simulink model "DCMotorControl"  (R2024b)
settings: Solver=VariableStepAuto  StartTime=0.0  StopTime=2  RelTol=1e-3
libraries: slpidlib x1
settings Model: Creator=chenitzhak6  LastModifiedBy=lenovo

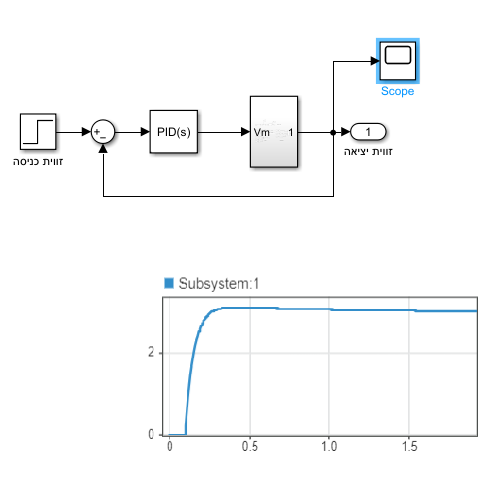
[thumbnail: Simulink's stored preview of the top-level diagram]
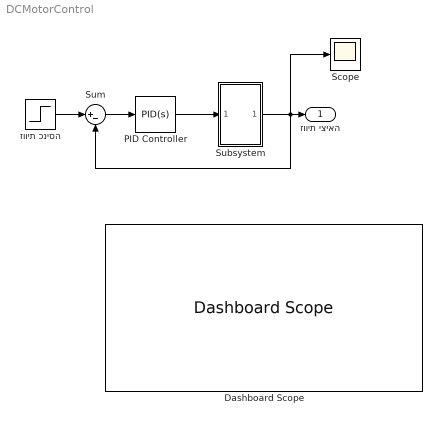
== system DCMotorControl ==
  Dashboard Scope : DashboardScope
  PID Controller : slpidlib/PID Controller  Controller=PID  Form=Parallel  TimeDomain=Continuous-time  UseExternalTs=off  SampleTime=-1  IntegratorMethod=Forward Euler  FilterMethod=Forward Euler  ControllerParametersSource=internal  P=1  I=1  UseKiTs=off  D=0  UseExternalDerivativeSource=off  N=100  UseFilter=on  TunerSelectOption=Transfer Function Based (PID Tuner App)  InitialConditionSource=internal  InitialConditionForIntegrator=0  InitialConditionForFilter=0  DifferentiatorICPrevScaledInput=0  ExternalReset=none  TrackingMode=off  Kt=1  LimitOutput=off  SatLimitsSource=internal  UpperSaturationLimit=inf  LowerSaturationLimit=-inf  LinearizeAsGain=on  AntiWindupMode=none  Kb=1  LimitIntegrator=off  UpperIntegratorSaturationLimit=inf  LowerIntegratorSaturationLimit=-inf  POutMin=[]  POutMax=[]  IOutMin=[]  IOutMax=[]  DOutMin=[]  DOutMax=[]  NOutMin=[]  NOutMax=[]  SumOutMin=[]  SumOutMax=[]  SaturationOutMin=[]  SaturationOutMax=[]  PParamMin=[]  PParamMax=[]  IParamMin=[]  IParamMax=[]  DParamMin=[]  DParamMax=[]  NParamMin=[]  NParamMax=[]  KbParamMin=[]  KbParamMax=[]  KtParamMin=[]  KtParamMax=[]  KbOutMin=[]  KbOutMax=[]  KtOutMin=[]  KtOutMax=[]  IntegratorOutMin=[]  IntegratorOutMax=[]  FilterOutMin=[]  FilterOutMax=[]  SumI1OutMin=[]  SumI1OutMax=[]  SumI2OutMin=[]  SumI2OutMax=[]  SumI3OutMin=[]  SumI3OutMax=[]  SumI4OutMin=[]  SumI4OutMax=[]  SumDOutMin=[]  SumDOutMax=[]  DifferentiatorOutMin=[]  DifferentiatorOutMax=[]  FilterDiffOutCoefMin=[]  FilterDiffOutCoefMax=[]  ReciprocalOutMin=[]  ReciprocalOutMax=[]  SumDenOutMin=[]  SumDenOutMax=[]  SumNumOutMin=[]  SumNumOutMax=[]  DivideOutMin=[]  DivideOutMax=[]  UdiffTsProdOutMin=[]  UdiffTsProdOutMax=[]  NTsProdOutMin=[]  NTsProdOutMax=[]  UintegralTsProdOutMin=[]  UintegralTsProdOutMax=[]  UngainTsProdOutMin=[]  UngainTsProdOutMax=[]  ClampingZeroOutDataTypeStr=Inherit: Inherit via back propagation  ClampingZeroOutMin=[]  ClampingZeroOutMax=[]  FilterDenConstantOutDataTypeStr=Inherit: Inherit via back propagation  FilterDenConstantOutMin=[]  FilterDenConstantOutMax=[]  PCopyOutDataTypeStr=Inherit: Inherit via back propagation  PCopyOutMin=[]  PCopyOutMax=[]  NCopyOutDataTypeStr=Inherit: Inherit via back propagation  NCopyOutMin=[]  NCopyOutMax=[]  IntegratorContinuousStateAttributes=''  IntegratorStateMustResolveToSignalObject=off  IntegratorRTWStateStorageClass=Auto  FilterContinuousStateAttributes=''  FilterStateMustResolveToSignalObject=off  FilterRTWStateStorageClass=Auto  ParallelPVariant=InternalParameters  IdealPVariant=Disabled  IVariant=InternalParameters  DVariant=InternalParameters  IntegratorVariant=Continuous  SatVariant=Disabled  AWVariant=Passthrough  PCopyVariant=Disabled  TRVariant=Disabled  FdbkBlocksVariant=Forward  IdealPFdbkVariant=Disabled  SatFdbkVariant=Disabled  DerivativeFilterVariant=ContFilter  NVariant=InternalParameters  NCopyVariant=Disabled  FilterICVariant=InternalICsFilter  IntegratorICVariant=InternalICs  ExternalResetVariant=Disabled  TRSumVariant=Passthrough  SumFdbkVariant=Disabled  SumVariant=Sum_PID  TsampFilterVariant=InternalTs  TsampNgainVariant=Passthrough  TsampIntegralVariant=Disabled_SignalSpec  ExternalSaturationOutDataTypeStr=Inherit: Same as second input  DerivativeSourceVariant=ErrorSignal  PreIntVariant=InternalPreInt
  Scope : Scope
  Subsystem : Subsystem
  Sum : Sum  Inputs=|+-
  זווית כניסה : Step  Time=0.1  After=3  SampleTime=0
  זווית יציאה : Outport
  wires:
  Subsystem/1(Out1) -> Scope/1, Sum/2, זווית יציאה/1
  PID Controller/1 -> Subsystem/1(Vm)
  זווית כניסה/1 -> Sum/1
  Sum/1 -> PID Controller/1

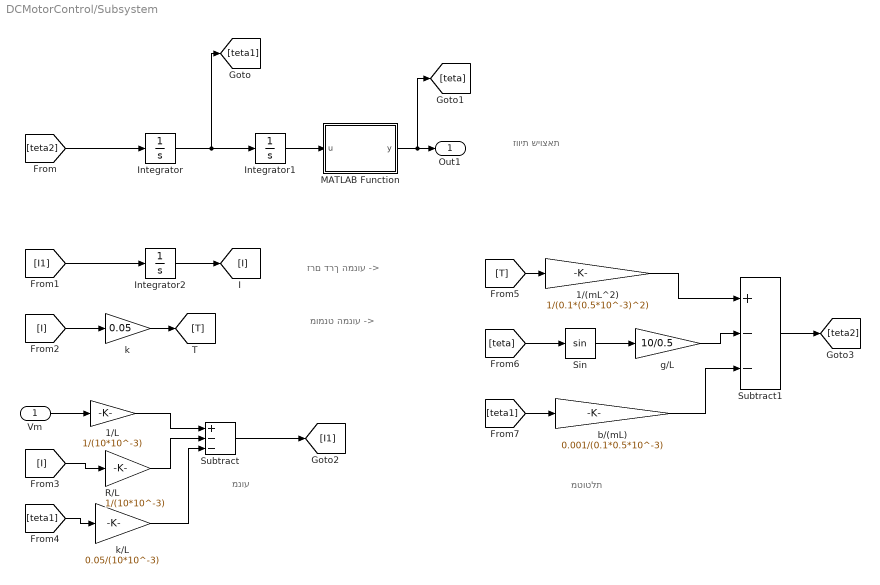
== system DCMotorControl/Subsystem ==
  note: מטוטלת
  note: מנוע
  note: זרם דרך המנוע ->
  note: מומנט המנוע ->
  note: זווית שיוצאת
  Vm : Inport
  1/(mL^2) : Gain  Gain=1/(0.1*(0.5*10^-3)^2)
  1/L : Gain  Gain=1/(10*10^-3)
  Integrator : Integrator
  Integrator1 : Integrator
  Integrator2 : Integrator
  MATLAB Function : MATLAB Function  TreatAsAtomicUnit=on
  R/L : Gain  Gain=1/(10*10^-3)
  Sin : Trigonometry
  Subtract : Sum  Inputs=+--
  Subtract1 : Sum  Inputs=+--
  b/(mL) : Gain  Gain=0.001/(0.1*0.5*10^-3)
  g/L : Gain  Gain=10/0.5
  k : Gain  Gain=0.05
  k/L : Gain  Gain=0.05/(10*10^-3)
  Out1 : Outport
  wires:
  b/(mL)/1 -> Subtract1/3
  Subtract1/1 -> [teta2]
  1/(mL^2)/1 -> Subtract1/1
  [I1] -> Integrator2/1
  Vm/1 -> 1/L/1
  Integrator/1 -> [teta1], Integrator1/1
  k/L/1 -> Subtract/3
  [teta] -> Sin/1
  [teta1] -> b/(mL)/1
  k/1 -> [T]
  Integrator2/1 -> [I]
  1/L/1 -> Subtract/1
  Integrator1/1 -> MATLAB Function/1(u)
  [I] -> R/L/1
  [I] -> k/1
  Sin/1 -> g/L/1
  R/L/1 -> Subtract/2
  g/L/1 -> Subtract1/2
  [teta2] -> Integrator/1
  [T] -> 1/(mL^2)/1
  [teta1] -> k/L/1
  Subtract/1 -> [I1]
  MATLAB Function/1(y) -> [teta], Out1/1

== matlab function DCMotorControl/Subsystem/MATLAB Function ==
  data: u input; y output
function y = fcn(u)
if(u>pi)
    u=mod(u,pi);
end
y = u;
